simulink model "car_simulation"  (R2019a)
settings: Solver=VariableStepAuto  StartTime=0.0  StopTime=3  RelTol=1e-3
values from neighbouring files (symbols this model uses):
  a = 2    [animation.m]
  b = 5    [animation.m]
undefined symbols (not defined in the file or in its folder): DiscIntNeverNeededParam
settings Model: Creator=ray  LastModifiedBy=ASUS
settings DebuggingCC: AlgebraicLoopMsg=none

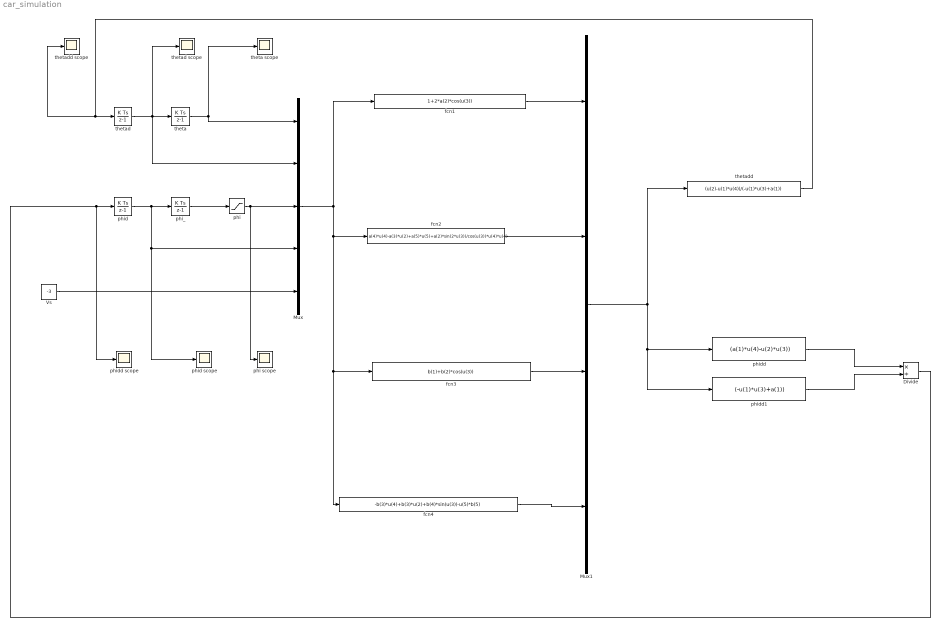
== system car_simulation ==
  Divide : Product  Inputs=*/
  Mux : Mux  Inputs=5
  Mux1 : Mux
  Vs : Constant  Value=-3
  fcn1 : Fcn  Expr=1+2*a(2)*cos(u(3))
  fcn2 : Fcn  Expr=a(4)*u(4)-a(3)*u(2)+a(5)*u(5)+a(2)*sin(2*u(3))/cos(u(3))*u(4)*u(4)
  fcn3 : Fcn  Expr=b(1)+b(2)*cos(u(3))
  fcn4 : Fcn  Expr=-b(3)*u(4)+b(3)*u(2)+b(4)*sin(u(3))-u(5)*b(5)
  phi : Saturate  UpperLimit=1.6  LowerLimit=-1.6
  "phi scope " : Scope
  phi_ : DiscreteIntegrator  SampleTime=0.01  ICPrevOutput=DiscIntNeverNeededParam  ICPrevScaledInput=DiscIntNeverNeededParam
  phid : DiscreteIntegrator  SampleTime=0.01  ICPrevOutput=DiscIntNeverNeededParam  ICPrevScaledInput=DiscIntNeverNeededParam
  "phid scope " : Scope
  phidd : Fcn  Expr=(a(1)*u(4)-u(2)*u(3))
  "phidd scope " : Scope
  phidd1 : Fcn  Expr=(-u(1)*u(3)+a(1))
  theta : DiscreteIntegrator  SampleTime=0.01  ICPrevOutput=DiscIntNeverNeededParam  ICPrevScaledInput=DiscIntNeverNeededParam
  theta scope : Scope
  thetad : DiscreteIntegrator  SampleTime=0.01  ICPrevOutput=DiscIntNeverNeededParam  ICPrevScaledInput=DiscIntNeverNeededParam
  "thetad scope " : Scope
  thetadd : Fcn  Expr=(u(2)-u(1)*u(4))/(-u(1)*u(3)+a(1))
  "thetadd scope " : Scope
  wires:
  phid/1 -> Mux/4, "phid scope "/1, phi_/1
  phi_/1 -> phi/1
  phi/1 -> Mux/3, "phi scope "/1
  Vs/1 -> Mux/5
  fcn4/1 -> Mux1/4
  fcn3/1 -> Mux1/3
  fcn2/1 -> Mux1/2
  fcn1/1 -> Mux1/1
  theta/1 -> theta scope/1, Mux/1
  Mux1/1 -> thetadd/1, phidd1/1, phidd/1
  Mux/1 -> fcn2/1, fcn3/1, fcn4/1, fcn1/1
  thetad/1 -> "thetad scope "/1, Mux/2, theta/1
  thetadd/1 -> "thetadd scope "/1, thetad/1
  phidd/1 -> Divide/1
  phidd1/1 -> Divide/2
  Divide/1 -> "phidd scope "/1, phid/1
